simulink model "sfuntest_gui"  (Simulink 7.2)
settings: Solver=FixedStepDiscrete  StartTime=0.0  StopTime=1  FixedStep=1/12  RelTol=1e-3
undefined symbols (not defined in the file or in its folder): init_aileron, init_elevator, init_flaps, init_gear, init_mixture, init_rudder, init_run_set, init_throttle
libraries: aerolibconvert2 x2
settings Model: Creator=Bri  LastModifiedBy=Bri

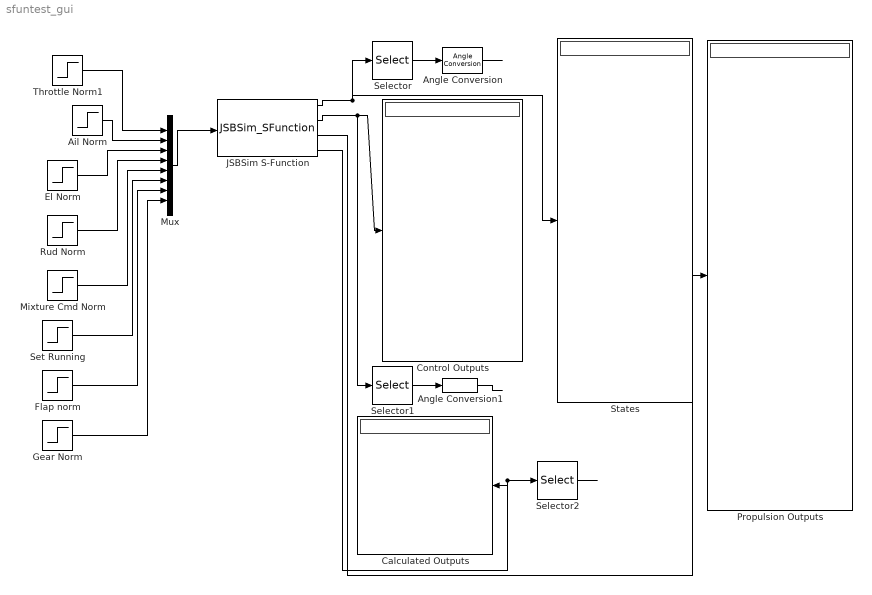
== system sfuntest_gui ==
  Ail Norm : Step  Time=3  Before=init_aileron  After=init_aileron  SampleTime=0
  Angle Conversion : aerolibconvert2/Angle Conversion  SystemSampleTime=-1  IU=rad  OU=deg
  Angle Conversion1 : aerolibconvert2/Angle Conversion  SystemSampleTime=-1  IU=rad  OU=deg
  Calculated Outputs : Display
  Control Outputs : Display
  El Norm : Step  Time=15  Before=init_elevator  After=init_elevator  SampleTime=0
  Flap norm : Step  Time=0  Before=init_flaps  After=init_flaps  SampleTime=0
  Gear Norm : Step  Time=0  Before=init_gear  After=init_gear  SampleTime=0
  JSBSim S-Function : S-Function  FunctionName=JSBSim_SFunction  Parameters=ac_name, IC_states, IC_controls, IC_delta_t, IC_verbosity,IC_sim_multiplier  EnableBusSupport=off  mask{ac_name='f16', IC_states=[ 399.9995 0 0 0 0 0 27887.34 122 34 0 0 0 ], IC_controls=[ 0.23296 0 -0.02 0 0.09 1 0 0 ], IC_delta_t=0.00833, IC_verbosity='debug', IC_sim_multiplier=13.96}
      mask prompts: ac_name "AC:"; IC_states "States:"; IC_controls "Controls:"; IC_delta_t "Delta:"; IC_verbosity "Verbosity:"; IC_sim_multiplier "JSBSim Multiplier:"
  Mixture Cmd Norm : Step  Time=.1  Before=init_mixture  After=init_mixture  SampleTime=0
  Mux : Mux  Inputs=8
  Propulsion Outputs : Display
  Rud Norm : Step  Time=5  Before=init_rudder  After=init_rudder  SampleTime=0
  Selector : Selector  InputPortWidth=19  IndexOptions=Index vector (dialog)  Indices=[5]  OutputSizes=1
  Selector1 : Selector  InputPortWidth=13  IndexOptions=Index vector (dialog)  Indices=2  OutputSizes=1
  Selector2 : Selector  InputPortWidth=7  IndexOptions=Index vector (dialog)  Indices=5  OutputSizes=1
  Set Running : Step  Time=0  Before=init_run_set  After=init_run_set  SampleTime=0
  States : Display
  Throttle Norm1 : Step  Time=0  Before=init_throttle  After=init_throttle  SampleTime=0
  wires:
  JSBSim S-Function/1 -> States/1, Selector/1
  Mux/1 -> JSBSim S-Function/1
  Throttle Norm1/1 -> Mux/1
  El Norm/1 -> Mux/3
  Selector/1 -> Angle Conversion/1
  Rud Norm/1 -> Mux/4
  Mixture Cmd Norm/1 -> Mux/5
  Set Running/1 -> Mux/6
  Flap norm/1 -> Mux/7
  Gear Norm/1 -> Mux/8
  JSBSim S-Function/2 -> Control Outputs/1, Selector1/1
  JSBSim S-Function/3 -> Propulsion Outputs/1
  JSBSim S-Function/4 -> Calculated Outputs/1, Selector2/1
  Angle Conversion/1 -> ?
  Selector1/1 -> Angle Conversion1/1
  Angle Conversion1/1 -> ?
  Ail Norm/1 -> Mux/2
  Selector2/1 -> ?
